simulink library "hvs_framelib_zfCetrax"  (R2016a)
settings: Solver=ode1  StartTime=0.0  StopTime=Inf  FixedStep=0.001  RelTol=1e-3
undefined symbols (not defined in the file): API1_dcac_efficiency, API2_dcac_efficiency, API3_dcac_efficiency, aux_power_flag, aux_power_selector_aux_power_flag, dcdc_effmap, dcdc_effmap_cooltemp_3rdD, dcdc_effmap_cur_2ndD, dcdc_effmap_vlt_1stD, DCL1_dcdc_effmap, DCL1_dcdc_effmap_cooltemp_3rdD, DCL1_dcdc_effmap_cur_2ndD, DCL1_dcdc_effmap_vlt_1stD
libraries: Electrical_to_Mechanical_gen x9, Electrical_converter x6, Electrical_to_Thermal_gen x3, Electrical_charger x3, Powernet x3, Enrg_conv_El_to_Mec_zfCetrax x3, ePTO x3, simulink x3
(part 2 of 2)

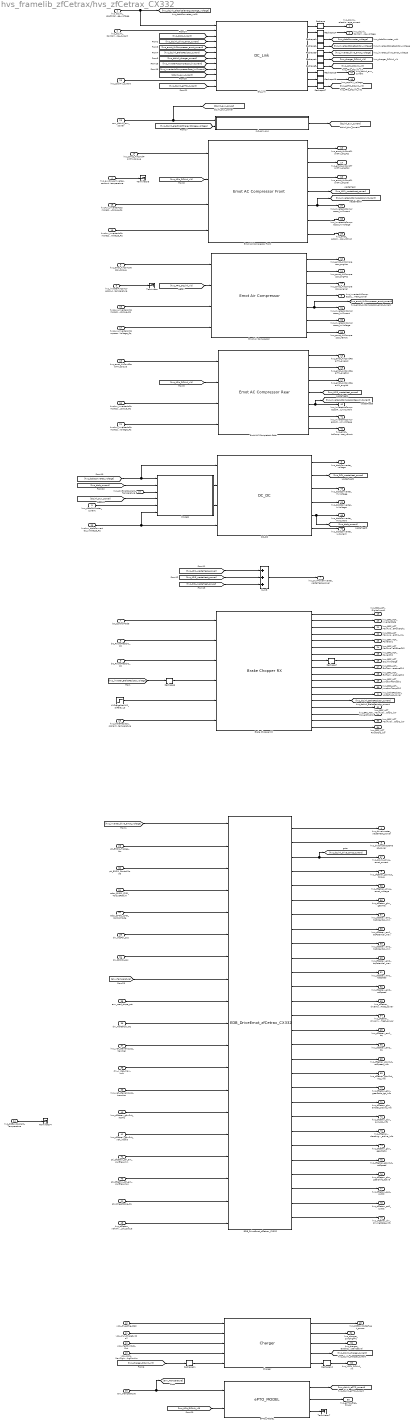
== system hvs_framelib_zfCetrax/hvs_zfCetrax_CX332 ==
  hvs_dcLink_electricalEnergyStorage_voltage : Inport
  hvs_dcLink_ControllableEnergySource_current : Inport  Port=2
  hvs_dcdcConverter_current : Inport  Port=3
  hvs_auxPowerInverter_coolant_temperature : Inport  Port=4
  hvs_inverterAirCompressor_coolant_temperature : Inport  Port=5
  hvs_emot_AirCompressor_torque : Inport  Port=6
  brc_ControlMode : Inport  Port=7
  brc_PowerReqCh1_kW : Inport  Port=8
  brc_PowerReqCh2_kW : Inport  Port=9
  vccu_PlugChrg_Stat : Inport  Port=10
  vccu_Pwr_ChargSysSoll : Inport  Port=11
  vccu_TestPwrSLQ_Out : Inport  Port=12
  vccu_CAN_MaxPlginChrgPwrLim : Inport  Port=13
  hvs_emot_AirCondFrontHV_torque : Inport  Port=14
  hvs_emot_AirCondRearHV_torque : Inport  Port=15
  hvsAux_InverterAirCompressor_torque_Rq : Inport  Port=16
  hvsAux_InverterAirCompressor_Voltage_Rq : Inport  Port=17
  hvsAux_InverterAcCompressorFront_torque_Rq : Inport  Port=18
  hvsAux_InverterAcCompressorFront_Voltage_Rq : Inport  Port=19
  hvsAux_InverterAcCompressorRear_torque_Rq : Inport  Port=20
  hvsAux_InverterAcCompressorRear_Voltage_Rq : Inport  Port=21
  hvsAux_dcdcConverter_LvVoltage_Rq : Inport  Port=22
  env_dcLink_aux_power : Inport  Port=23
  hvs_DCBoxCoolant_Temperature : Inport  Port=24
  hvs_coolHV_current : Inport  Port=25
  env_Temperature : Inport  Port=26
  hvs_drvEmotCoolant_Temperature : Inport  Port=27
  hvs_brakeResistor_coolant_temperature : Inport  Port=28
  pti_EMD1_TrqReq_Nm : Inport  Port=29
  pti_EMD1_ControlMode : Inport  Port=30
  edcu_EMD1_CMD_TorqueRefLim : Inport  Port=31
  edcu_EMD1_CMD_ControlMode : Inport  Port=32
  drv_AccPdl_pos : Inport  Port=33
  drv_BrkPdl_pos : Inport  Port=34
  env_road_slope_pct : Inport  Port=35
  drv_HaltBrkSw_Rq : Inport  Port=36
  hvs_veh_GenericLoss_transVel : Inport  Port=37
  drv_v_des_max_kmh : Inport  Port=38
  hvs_veh_GenericLoss_transAcc : Inport  Port=39
  hvs_zfCetrax_gbxOut_resTrq : Inport  Port=40
  hvs_zfCetrax_gbxOut_veh_inertia : Inport  Port=41
  pti_zfCetrax_ctrl_em_pwrElec_min : Inport  Port=42
  pti_zfCetrax_ctrl_em_pwrElec_max : Inport  Port=43
  pti_WheelBrake_trq : Inport  Port=44
  hvs_zfCetrax_vehWheel_brk_torque : Inport  Port=45
  Brake Chopper RX : Electrical_to_Thermal_gen/Brake Chopper RX
  Charger : Electrical_charger/Charger
  DC_DC : Electrical_converter/DC_DC
  DC_Link : Powernet/DC_Link
  EDB_DriveEmot_zfCetrax_CX332 : Enrg_conv_El_to_Mec_zfCetrax/EDB_DriveEmot_zfCetrax_CX332
  Emot AC Compressor Front : Electrical_to_Mechanical_gen/Emot AC Compressor Front
  Emot AC Compressor Rear : Electrical_to_Mechanical_gen/Emot AC Compressor Rear
  Emot Air Compressor : Electrical_to_Mechanical_gen/Emot Air Compressor
  HVFreigabeHW2_SiRelay_D : Step  Time=5.502  SampleTime=0
  Process : Subsystem
  Reshape{,1..7,11..12,14..17} (14 alike) : Reshape
  Sum8 : Sum  Inputs=+++  SaturateOnIntegerOverflow=on  InputSameDT=on  OutDataTypeStr=Inherit: Same as first input
  Terminator{,4..5,7} (4 alike) : Terminator
  ePTO_MODEL : ePTO/ePTO_MODEL
  sub_env_aux : Subsystem
  hvs_dcLink_electricalEnergyStorage_current : Outport
  hvs_dcLink_ControllableEnergySource_voltage : Outport  Port=2
  hvs_dcdcConverter_voltage : Outport  Port=3
  hvs_driveInverter_wasteHeat_power : Outport  Port=4
  hvs_drvEmotWasteHeat_power : Outport  Port=5
  hvs_brakeResistor_wasteHeat_power : Outport  Port=6
  hvs_auxPowerInverter_wasteHeat_power : Outport  Port=7
  hvs_inverterAirCompressor_wasteHeat_power : Outport  Port=8
  hvs_zfCetrax_gbxOut_torque : Outport  Port=9
  hvs_emot_AirCompressor_angAcc : Outport  Port=10
  hvs_emot_AirCompressor_angPos : Outport  Port=11
  hvs_emot_AirCompressor_angVel : Outport  Port=12
  hvs_emot_AirCondFrontHV_angAcc : Outport  Port=13
  hvs_emot_AirCondFrontHV_angPos : Outport  Port=14
  hvs_emot_AirCondFrontHV_angVel : Outport  Port=15
  hvs_emot_AirCondRearHV_angAcc : Outport  Port=16
  hvs_emot_AirCondRearHV_angVel : Outport  Port=17
  hvs_emot_AirCondRearHV_angPos : Outport  Port=18
  hvs_BRC_ACT_DigitalInput1 : Outport  Port=19
  hvs_BRC_ACT_InverterState : Outport  Port=20
  hvs_BRC_ACT_MaxAvailablePowerCh1 : Outport  Port=21
  hvs_BRC_ACT_MaxAvailablePowerCh1_VAL : Outport  Port=22
  hvs_BRC_ACT_PowerCh1 : Outport  Port=23
  hvs_BRC_ACT_MaxAvailablePowerCh2 : Outport  Port=24
  hvs_BRC_ACT_PowerCh2 : Outport  Port=25
  hvs_BRC_ACT_DcLinkVoltage : Outport  Port=26
  hvs_BRC_ACT_ExtTemperatureCh1 : Outport  Port=27
  hvs_BRC_ACT_ExtTemperatureCh2 : Outport  Port=28
  hvs_BRC_ACT_JunctionTempCh1 : Outport  Port=29
  hvs_BRC_ACT_JunctionTempCh2 : Outport  Port=30
  hvs_charger_pwrChrgPhy : Outport  Port=31
  hvs_charger_ExtChrgr_Isolation_ResistanceCval : Outport  Port=32
  hvs_VCCU_DCLink_vlt : Outport  Port=33
  hvs_InverterAirCompressor_hvCurrent : Outport  Port=34
  hvs_InverterAirCompressor_hvVoltage : Outport  Port=35
  hvs_emot_AirCompressor_nEmot : Outport  Port=36
  hvs_InverterAcCompressor_hvCurrent : Outport  Port=37
  hvs_InverterAcCompressor_hvVoltage : Outport  Port=38
  hvs_emot_AcCompressor_nEmot : Outport  Port=39
  hvs_InverterAcCompressorRear_hvCurrent : Outport  Port=40
  hvs_InverterAcCompressorRear_hvVoltage : Outport  Port=41
  hvs_emot_AcCompressorRear_nEmot : Outport  Port=42
  hvs_dcdcConverter_HvVoltage : Outport  Port=43
  hvs_dcdcConverter_LvVoltage : Outport  Port=44
  hvs_dcdcConverter_HvCurrent : Outport  Port=45
  hvs_dcdcConverter_LvCurrent : Outport  Port=46
  hvs_dcLink_aux_current : Outport  Port=47
  hvs_DCBoxWasteHeat_power : Outport  Port=48
  hvs_coolHV_voltage : Outport  Port=49
  hvs_ePTO_Elec_Power : Outport  Port=50
  hvs_BRC_ACT_MaxAvailablePowerCh1_kW : Outport  Port=51
  hvs_BRC_ACT_PowerCh1_kW : Outport  Port=52
  hvs_BRC_ACT_MaxAvailablePowerCh2_kW : Outport  Port=53
  hvs_BRC_ACT_PowerCh2_kW : Outport  Port=54
  hvs_zfCetrax_drive_emot_voltage : Outport  Port=55
  hvs_zfCetrax_gbx_gearAct : Outport  Port=56
  hvs_zfCetrax_em1_trqPotential_min : Outport  Port=57
  hvs_zfCetrax_em1_trqPotential_max : Outport  Port=58
  hvs_zfCetrax_em2_trqPotential_min : Outport  Port=59
  hvs_zfCetrax_em2_trqPotential_max : Outport  Port=60
  hvs_zfCetrax_em1_rotSpeed : Outport  Port=61
  hvs_zfCetrax_em2_rotSpeed : Outport  Port=62
  hvs_zfCetrax_drvEmotWasteHeat_power : Outport  Port=63
  hvs_zfCetrax_driveInverterWasteHeat_power : Outport  Port=64
  hvs_zfCetrax_em1_trq : Outport  Port=65
  hvs_zfCetrax_em2_trq : Outport  Port=66
  hvs_dcLink_drive_emot_current : Outport  Port=67
  hvs_zfCetrax_gbxOut_rotSpeed_info : Outport  Port=68
  hvs_zfCetrax_gbxOut_Acc_info : Outport  Port=69
  hvs_zfCetrax_gbx_gearRatio_tgt_info : Outport  Port=70
  hvs_zfCetrax_gbx_emDec_active_info : Outport  Port=71
  hvs_zfCetrax_gbx_pwrLoss_info : Outport  Port=72
  hvs_zfCetrax_derating_active_info : Outport  Port=73
  hvs_zfCetrax_gbx_gearRatio : Outport  Port=74
  hvs_zfCetrax_gbxOut_rotSpeed : Outport  Port=75
  hvs_zfCetrax_gbx_gearShift_active : Outport  Port=76
  hvs_zfCetrax_pe1_curDC : Outport  Port=77
  hvs_zfCetrax_pe2_curDC : Outport  Port=78
  hvs_zfCetrax_drv_drivingState_info : Outport  Port=79
  wires:
  EDB_DriveEmot_zfCetrax_CX332/28 -> hvs_zfCetrax_drv_drivingState_info/1
  Process/2(hvs_dcdcConv_current1) -> DC_DC/3
  Process/1(dcdc_conv_eff) -> DC_DC/2
  hvs_dcdcConverter_current/1 -> Process/5(hvs_dcdcConv_current)
  [dcLink_aux_power] -> Process/4(dcLink_aux_power)  "dcLink_aux_power"
  hvs_drvEmotCoolant_Temperature/1 -> Process/3(hvs_drvEmotCoolant_Temperature)
  [hvs_dcdc_current] -> Process/2(hvs_dcdc_HvCurrent)  "hvs_dcdc_HvCurrent"
  [hvs_dcLink_ePTO_current] -> DC_Link/12
  [hvs_APIs_DCLink_vlt] -> ePTO_MODEL/2
  ePTO_MODEL/3 -> Terminator7/1
  ePTO_MODEL/2 -> hvs_ePTO_Elec_Power/1
  ePTO_MODEL/1 -> [hvs_dcLink_ePTO_current]
  DC_Link/10 -> Reshape17/1
  Reshape17/1 -> [hvs_ePTO_DCLink_vlt]
  env_Temperature/1 -> [env_Temperature], ePTO_MODEL/1
  hvs_DCBoxCoolant_Temperature/1 -> Terminator4/1
  Charger/1 -> hvs_DCBoxWasteHeat_power/1  "hvs_DCBoxWasteHeat_power"
  hvsAux_dcdcConverter_LvVoltage_Rq/1 -> DC_DC/4, Process/6(hvsAux_dcdcConv_LvVoltage_Rq)  "hvsAux_dcdcConverter_LvVoltage_Rq"
  DC_Link/8 -> Reshape15/1
  [hvs_dcLink_electricalEnergyStorage_voltage] -> sub_env_aux/2(Nebenagg_voltage)
  sub_env_aux/1(dcLink_aux_current) -> [dcLink_aux_current]
  env_dcLink_aux_power/1 -> sub_env_aux/1(env_dcLink_aux_power), [dcLink_aux_power]
  [dcLink_aux_current] -> DC_Link/10
  Reshape12/1 -> hvs_VCCU_DCLink_vlt/1
  Reshape11/1 -> Charger/5
  Reshape7/1 -> hvs_BRC_ACT_DcLinkVoltage/1
  Reshape6/1 -> Brake Chopper RX/4
  Reshape5/1 -> [hvs_APIs_DCLink_vlt]
  Reshape4/1 -> [hvs_charger_DCLink_vlt]
  Reshape3/1 -> [hvs_inverter_drive_emot_voltage]
  Reshape2/1 -> [hvs_inverter_BrakeResistor_voltage]
  Reshape1/1 -> [hvs_dcdcConverter_voltage]
  Reshape/1 -> hvs_dcLink_electricalEnergyStorage_current/1
  [hvs_dcdc_current] -> DC_Link/3
  [hvs_DCL_wasteHeat_power] -> Sum8/3
  [hvs_API3_wasteHeat_power] -> Sum8/2
  [hvs_API1_wasteHeat_power] -> Sum8/1
  Sum8/1 -> hvs_auxPowerInverter_wasteHeat_power/1
  DC_DC/6 -> hvs_dcdcConverter_LvCurrent/1
  DC_DC/5 -> hvs_dcdcConverter_HvCurrent/1, [hvs_dcdc_current]
  DC_DC/4 -> hvs_dcdcConverter_LvVoltage/1
  DC_DC/3 -> hvs_dcdcConverter_HvVoltage/1
  DC_Link/3 -> Reshape1/1
  DC_DC/1 -> hvs_dcdcConverter_voltage/1
  DC_DC/2 -> [hvs_DCL_wasteHeat_power]
  [hvs_dcdcConverter_voltage] -> Process/1(hvs_dcdcConverter_voltage), DC_DC/1  "hvs_dcdcConverter_voltage"
  Emot AC Compressor Rear/4 -> [hvs_API3_wasteHeat_power]
  Emot AC Compressor Rear/5 -> hvs_InverterAcCompressorRear_hvCurrent/1, [hvs_InverterAcCompressorRear_hvCurrent]
  Emot AC Compressor Rear/6 -> hvs_InverterAcCompressorRear_hvVoltage/1
  Emot AC Compressor Rear/7 -> hvs_emot_AcCompressorRear_nEmot/1
  Emot AC Compressor Rear/2 -> hvs_emot_AirCondRearHV_angPos/1
  Emot AC Compressor Rear/3 -> hvs_emot_AirCondRearHV_angVel/1
  Emot AC Compressor Rear/1 -> hvs_emot_AirCondRearHV_angAcc/1
  hvsAux_InverterAcCompressorRear_Voltage_Rq/1 -> Emot AC Compressor Rear/4
  hvsAux_InverterAcCompressorRear_torque_Rq/1 -> Emot AC Compressor Rear/3
  [hvs_APIs_DCLink_vlt] -> Emot AC Compressor Rear/2
  hvs_emot_AirCondRearHV_torque/1 -> Emot AC Compressor Rear/1
  Emot AC Compressor Front/4 -> [hvs_API1_wasteHeat_power]
  Emot AC Compressor Front/6 -> hvs_InverterAcCompressor_hvVoltage/1
  Emot AC Compressor Front/7 -> hvs_emot_AcCompressor_nEmot/1
  Emot AC Compressor Front/3 -> hvs_emot_AirCondFrontHV_angVel/1
  Emot AC Compressor Front/2 -> hvs_emot_AirCondFrontHV_angPos/1
  Emot AC Compressor Front/1 -> hvs_emot_AirCondFrontHV_angAcc/1
  hvsAux_InverterAcCompressorFront_Voltage_Rq/1 -> Emot AC Compressor Front/4
  hvsAux_InverterAcCompressorFront_torque_Rq/1 -> Emot AC Compressor Front/3
  hvs_emot_AirCondFrontHV_torque/1 -> Emot AC Compressor Front/1
  [hvs_APIs_DCLink_vlt] -> Emot AC Compressor Front/2
  hvs_auxPowerInverter_coolant_temperature/1 -> Terminator5/1
  hvs_inverterAirCompressor_coolant_temperature/1 -> Terminator/1
  hvsAux_InverterAirCompressor_Voltage_Rq/1 -> Emot Air Compressor/4
  hvsAux_InverterAirCompressor_torque_Rq/1 -> Emot Air Compressor/3
  [hvs_APIs_DCLink_vlt] -> Emot Air Compressor/2
  DC_Link/7 -> Reshape5/1
  Emot Air Compressor/6 -> hvs_InverterAirCompressor_hvVoltage/1
  Emot Air Compressor/7 -> hvs_emot_AirCompressor_nEmot/1
  Emot Air Compressor/5 -> [hvs_emot_AirCompressor_emot_current], hvs_InverterAirCompressor_hvCurrent/1
  Emot Air Compressor/4 -> hvs_inverterAirCompressor_wasteHeat_power/1
  Emot Air Compressor/3 -> hvs_emot_AirCompressor_angVel/1
  Emot Air Compressor/2 -> hvs_emot_AirCompressor_angPos/1
  Emot Air Compressor/1 -> hvs_emot_AirCompressor_angAcc/1
  hvs_emot_AirCompressor_torque/1 -> Emot Air Compressor/1
  DC_Link/1 -> Reshape/1
  DC_Link/2 -> Reshape14/1
  hvs_dcLink_electricalEnergyStorage_voltage/1 -> [hvs_dcLink_electricalEnergyStorage_voltage], DC_Link/1
  hvs_dcLink_ControllableEnergySource_current/1 -> DC_Link/2
  DC_Link/4 -> Reshape2/1
  Brake Chopper RX/1 -> hvs_BRC_ACT_DigitalInput1/1
  Brake Chopper RX/2 -> hvs_BRC_ACT_InverterState/1
  Brake Chopper RX/3 -> hvs_BRC_ACT_MaxAvailablePowerCh1/1
  Brake Chopper RX/4 -> hvs_BRC_ACT_MaxAvailablePowerCh1_VAL/1
  Brake Chopper RX/5 -> hvs_BRC_ACT_PowerCh1/1
  Brake Chopper RX/6 -> hvs_BRC_ACT_MaxAvailablePowerCh2/1
  Brake Chopper RX/7 -> hvs_BRC_ACT_PowerCh2/1
  Brake Chopper RX/8 -> Reshape7/1
  Brake Chopper RX/9 -> hvs_BRC_ACT_ExtTemperatureCh1/1
  Brake Chopper RX/10 -> hvs_BRC_ACT_ExtTemperatureCh2/1
  Brake Chopper RX/11 -> hvs_BRC_ACT_JunctionTempCh1/1
  Brake Chopper RX/12 -> hvs_BRC_ACT_JunctionTempCh2/1
  [hvs_inverter_BrakeResistor_voltage] -> Reshape6/1
  DC_Link/5 -> Reshape3/1
  [hvs_dcLink_drive_emot_current] -> DC_Link/4
  [hvs_emot_AirCompressor_emot_current] -> DC_Link/5
  Brake Chopper RX/13 -> hvs_brakeResistor_wasteHeat_power/1
  Brake Chopper RX/14 -> [hvs_dcLink_BrakeResistor_current]
  [hvs_dcLink_BrakeResistor_current] -> DC_Link/6
  vccu_CAN_MaxPlginChrgPwrLim/1 -> Charger/4
  [hvs_charger_DCLink_vlt] -> Reshape11/1
  vccu_TestPwrSLQ_Out/1 -> Charger/3
  vccu_Pwr_ChargSysSoll/1 -> Charger/2
  vccu_PlugChrg_Stat/1 -> Charger/1
  Charger/2 -> hvs_charger_pwrChrgPhy/1
  Charger/3 -> hvs_charger_ExtChrgr_Isolation_ResistanceCval/1
  Charger/4 -> [hvs_dcLink_charger_current]
  [hvs_dcLink_charger_current] -> DC_Link/7
  DC_Link/6 -> Reshape4/1
  Charger/5 -> Reshape12/1
  Emot AC Compressor Front/5 -> [hvs_InverterAcCompressor_hvCurrent], hvs_InverterAcCompressor_hvCurrent/1
  [hvs_InverterAcCompressor_hvCurrent] -> DC_Link/8
  [hvs_InverterAcCompressorRear_hvCurrent] -> DC_Link/9
  Reshape14/1 -> hvs_dcLink_ControllableEnergySource_voltage/1
  Reshape15/1 -> hvs_dcLink_aux_current/1
  DC_Link/9 -> Reshape16/1
  Reshape16/1 -> hvs_coolHV_voltage/1
  hvs_coolHV_current/1 -> DC_Link/11
  HVFreigabeHW2_SiRelay_D/1 -> Brake Chopper RX/5
  brc_ControlMode/1 -> Brake Chopper RX/1
  brc_PowerReqCh1_kW/1 -> Brake Chopper RX/2
  brc_PowerReqCh2_kW/1 -> Brake Chopper RX/3
  hvs_brakeResistor_coolant_temperature/1 -> Brake Chopper RX/6
  Brake Chopper RX/15 -> hvs_BRC_ACT_MaxAvailablePowerCh1_kW/1
  Brake Chopper RX/16 -> hvs_BRC_ACT_PowerCh1_kW/1
  Brake Chopper RX/17 -> hvs_BRC_ACT_MaxAvailablePowerCh2_kW/1
  Brake Chopper RX/18 -> hvs_BRC_ACT_PowerCh2_kW/1
  [hvs_inverter_drive_emot_voltage] -> EDB_DriveEmot_zfCetrax_CX332/1
  pti_EMD1_TrqReq_Nm/1 -> EDB_DriveEmot_zfCetrax_CX332/2
  pti_EMD1_ControlMode/1 -> EDB_DriveEmot_zfCetrax_CX332/3
  edcu_EMD1_CMD_TorqueRefLim/1 -> EDB_DriveEmot_zfCetrax_CX332/4
  edcu_EMD1_CMD_ControlMode/1 -> EDB_DriveEmot_zfCetrax_CX332/5
  drv_AccPdl_pos/1 -> EDB_DriveEmot_zfCetrax_CX332/6
  drv_BrkPdl_pos/1 -> EDB_DriveEmot_zfCetrax_CX332/7
  [env_Temperature] -> EDB_DriveEmot_zfCetrax_CX332/8
  env_road_slope_pct/1 -> EDB_DriveEmot_zfCetrax_CX332/9
  drv_HaltBrkSw_Rq/1 -> EDB_DriveEmot_zfCetrax_CX332/10
  hvs_veh_GenericLoss_transVel/1 -> EDB_DriveEmot_zfCetrax_CX332/11
  drv_v_des_max_kmh/1 -> EDB_DriveEmot_zfCetrax_CX332/12
  hvs_veh_GenericLoss_transAcc/1 -> EDB_DriveEmot_zfCetrax_CX332/13
  hvs_zfCetrax_gbxOut_resTrq/1 -> EDB_DriveEmot_zfCetrax_CX332/14
  hvs_zfCetrax_gbxOut_veh_inertia/1 -> EDB_DriveEmot_zfCetrax_CX332/15
  pti_zfCetrax_ctrl_em_pwrElec_min/1 -> EDB_DriveEmot_zfCetrax_CX332/16
  pti_zfCetrax_ctrl_em_pwrElec_max/1 -> EDB_DriveEmot_zfCetrax_CX332/17
  EDB_DriveEmot_zfCetrax_CX332/3 -> hvs_dcLink_drive_emot_current/1, [hvs_dcLink_drive_emot_current]
  EDB_DriveEmot_zfCetrax_CX332/1 -> hvs_driveInverter_wasteHeat_power/1
  EDB_DriveEmot_zfCetrax_CX332/2 -> hvs_drvEmotWasteHeat_power/1
  EDB_DriveEmot_zfCetrax_CX332/4 -> hvs_zfCetrax_gbxOut_torque/1
  EDB_DriveEmot_zfCetrax_CX332/5 -> hvs_zfCetrax_drive_emot_voltage/1
  EDB_DriveEmot_zfCetrax_CX332/6 -> hvs_zfCetrax_gbx_gearAct/1
  EDB_DriveEmot_zfCetrax_CX332/7 -> hvs_zfCetrax_em1_trqPotential_min/1
  EDB_DriveEmot_zfCetrax_CX332/8 -> hvs_zfCetrax_em1_trqPotential_max/1
  EDB_DriveEmot_zfCetrax_CX332/9 -> hvs_zfCetrax_em2_trqPotential_min/1
  EDB_DriveEmot_zfCetrax_CX332/10 -> hvs_zfCetrax_em2_trqPotential_max/1
  EDB_DriveEmot_zfCetrax_CX332/11 -> hvs_zfCetrax_em1_rotSpeed/1
  EDB_DriveEmot_zfCetrax_CX332/12 -> hvs_zfCetrax_em2_rotSpeed/1
  EDB_DriveEmot_zfCetrax_CX332/13 -> hvs_zfCetrax_drvEmotWasteHeat_power/1
  EDB_DriveEmot_zfCetrax_CX332/14 -> hvs_zfCetrax_driveInverterWasteHeat_power/1
  EDB_DriveEmot_zfCetrax_CX332/15 -> hvs_zfCetrax_em1_trq/1
  EDB_DriveEmot_zfCetrax_CX332/16 -> hvs_zfCetrax_em2_trq/1
  pti_WheelBrake_trq/1 -> EDB_DriveEmot_zfCetrax_CX332/18
  EDB_DriveEmot_zfCetrax_CX332/17 -> hvs_zfCetrax_gbxOut_rotSpeed_info/1
  EDB_DriveEmot_zfCetrax_CX332/18 -> hvs_zfCetrax_gbxOut_Acc_info/1
  EDB_DriveEmot_zfCetrax_CX332/19 -> hvs_zfCetrax_gbx_gearRatio_tgt_info/1
  EDB_DriveEmot_zfCetrax_CX332/20 -> hvs_zfCetrax_gbx_emDec_active_info/1
  EDB_DriveEmot_zfCetrax_CX332/21 -> hvs_zfCetrax_gbx_pwrLoss_info/1
  EDB_DriveEmot_zfCetrax_CX332/22 -> hvs_zfCetrax_derating_active_info/1
  EDB_DriveEmot_zfCetrax_CX332/23 -> hvs_zfCetrax_gbx_gearRatio/1
  hvs_zfCetrax_vehWheel_brk_torque/1 -> EDB_DriveEmot_zfCetrax_CX332/19
  EDB_DriveEmot_zfCetrax_CX332/24 -> hvs_zfCetrax_gbxOut_rotSpeed/1
  EDB_DriveEmot_zfCetrax_CX332/25 -> hvs_zfCetrax_gbx_gearShift_active/1
  EDB_DriveEmot_zfCetrax_CX332/26 -> hvs_zfCetrax_pe1_curDC/1
  EDB_DriveEmot_zfCetrax_CX332/27 -> hvs_zfCetrax_pe2_curDC/1

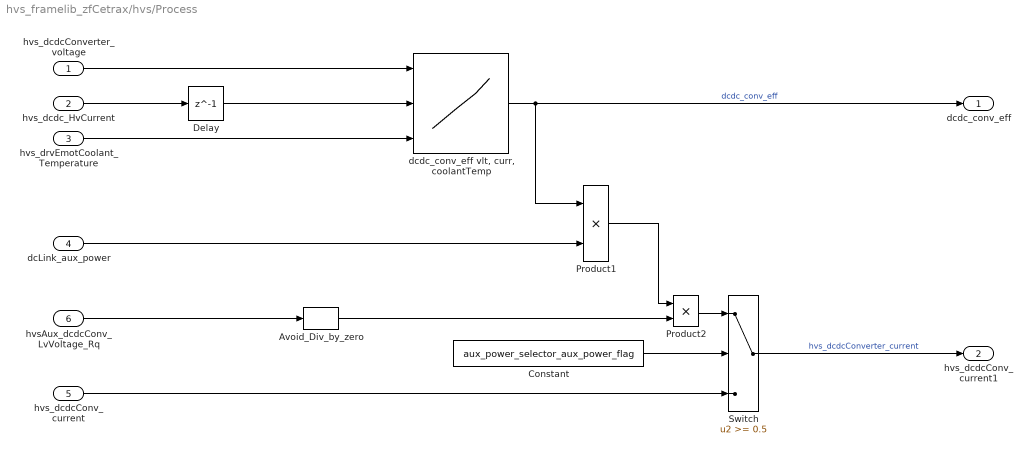
== system hvs_framelib_zfCetrax/hvs/Process ==
  hvs_dcdcConverter_voltage : Inport
  hvs_dcdc_HvCurrent : Inport  Port=2
  hvs_drvEmotCoolant_Temperature : Inport  Port=3
  dcLink_aux_power : Inport  Port=4
  hvs_dcdcConv_current : Inport  Port=5
  hvsAux_dcdcConv_LvVoltage_Rq : Inport  Port=6
  Avoid_Div_by_zero : Electrical_converter/DC_DC/Avoid_Div_by_zero
  Constant : Constant  Value=aux_power_selector_aux_power_flag
  Delay : Delay  DelayLength=1  InitialCondition=0
  Product1 : Product  Inputs=**  RndMeth=Zero
  Product2 : Product  Inputs=**  RndMeth=Zero
  Switch : Switch  Threshold=0.5
  "dcdc_conv_eff vlt, curr, coolantTemp" : Lookup_n-D  NumberOfTableDimensions=3  BreakpointsForDimension1=DCL1_dcdc_effmap_vlt_1stD  BreakpointsForDimension2=DCL1_dcdc_effmap_cur_2ndD  BreakpointsForDimension3=DCL1_dcdc_effmap_cooltemp_3rdD  Table=DCL1_dcdc_effmap  ExtrapMethod=Clip  RndMeth=Simplest  InputSameDT=on
  dcdc_conv_eff : Outport
  hvs_dcdcConv_current1 : Outport  Port=2
  wires:
  Delay/1 -> "dcdc_conv_eff vlt, curr, coolantTemp"/2
  hvs_dcdc_HvCurrent/1 -> Delay/1
  "dcdc_conv_eff vlt, curr, coolantTemp"/1 -> dcdc_conv_eff/1, Product1/1  "dcdc_conv_eff"
  Product2/1 -> Switch/1
  Product1/1 -> Product2/1
  hvs_dcdcConv_current/1 -> Switch/3
  Switch/1 -> hvs_dcdcConv_current1/1  "hvs_dcdcConverter_current"
  dcLink_aux_power/1 -> Product1/2
  Avoid_Div_by_zero/1 -> Product2/2
  Constant/1 -> Switch/2
  hvsAux_dcdcConv_LvVoltage_Rq/1 -> Avoid_Div_by_zero/1
  hvs_dcdcConverter_voltage/1 -> "dcdc_conv_eff vlt, curr, coolantTemp"/1
  hvs_drvEmotCoolant_Temperature/1 -> "dcdc_conv_eff vlt, curr, coolantTemp"/3

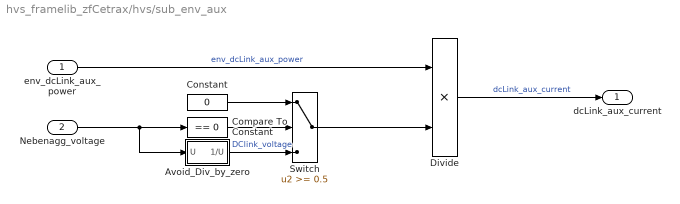
== system hvs_framelib_zfCetrax/hvs/sub_env_aux ==
  env_dcLink_aux_power : Inport
  Nebenagg_voltage : Inport  Port=2
  Avoid_Div_by_zero : Subsystem
  Compare To Constant : simulink/Logic and Bit Operations/Compare To Constant  relop===  const=0  OutDataTypeStr=boolean
  Constant : Constant  Value=0
  Divide : Product
  Switch : Switch  Threshold=0.5
  dcLink_aux_current : Outport
  wires:
  Divide/1 -> dcLink_aux_current/1  "dcLink_aux_current"
  Nebenagg_voltage/1 -> Avoid_Div_by_zero/1(U), Compare To Constant/1
  Avoid_Div_by_zero/1(1/U) -> Switch/3  "DClink_voltage"
  env_dcLink_aux_power/1 -> Divide/1  "env_dcLink_aux_power"
  Compare To Constant/1 -> Switch/2
  Constant/1 -> Switch/1
  Switch/1 -> Divide/2

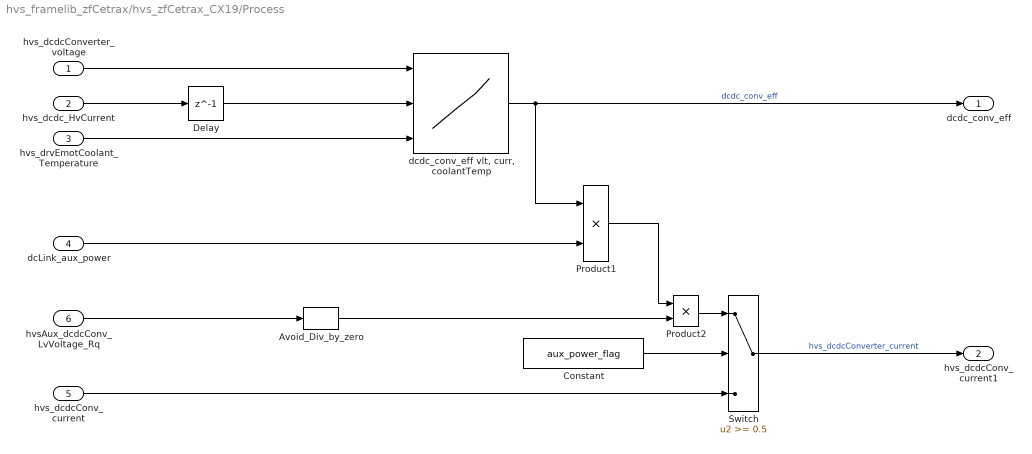
== system hvs_framelib_zfCetrax/hvs_zfCetrax_CX19/Process ==
  hvs_dcdcConverter_voltage : Inport
  hvs_dcdc_HvCurrent : Inport  Port=2
  hvs_drvEmotCoolant_Temperature : Inport  Port=3
  dcLink_aux_power : Inport  Port=4
  hvs_dcdcConv_current : Inport  Port=5
  hvsAux_dcdcConv_LvVoltage_Rq : Inport  Port=6
  Avoid_Div_by_zero : Electrical_converter/DC_DC/Avoid_Div_by_zero
  Constant : Constant  Value=aux_power_flag
  Delay : Delay  DelayLength=1  InitialCondition=0
  Product1 : Product  Inputs=**  RndMeth=Zero
  Product2 : Product  Inputs=**  RndMeth=Zero
  Switch : Switch  Threshold=0.5
  "dcdc_conv_eff vlt, curr, coolantTemp" : Lookup_n-D  NumberOfTableDimensions=3  BreakpointsForDimension1=dcdc_effmap_vlt_1stD  BreakpointsForDimension2=dcdc_effmap_cur_2ndD  BreakpointsForDimension3=dcdc_effmap_cooltemp_3rdD  Table=dcdc_effmap  ExtrapMethod=Clip  RndMeth=Simplest  InputSameDT=on
  dcdc_conv_eff : Outport
  hvs_dcdcConv_current1 : Outport  Port=2
  wires:
  hvs_drvEmotCoolant_Temperature/1 -> "dcdc_conv_eff vlt, curr, coolantTemp"/3
  hvs_dcdcConverter_voltage/1 -> "dcdc_conv_eff vlt, curr, coolantTemp"/1
  hvsAux_dcdcConv_LvVoltage_Rq/1 -> Avoid_Div_by_zero/1
  Constant/1 -> Switch/2
  Avoid_Div_by_zero/1 -> Product2/2
  dcLink_aux_power/1 -> Product1/2
  Switch/1 -> hvs_dcdcConv_current1/1  "hvs_dcdcConverter_current"
  hvs_dcdcConv_current/1 -> Switch/3
  Product1/1 -> Product2/1
  Product2/1 -> Switch/1
  "dcdc_conv_eff vlt, curr, coolantTemp"/1 -> Product1/1, dcdc_conv_eff/1  "dcdc_conv_eff"
  hvs_dcdc_HvCurrent/1 -> Delay/1
  Delay/1 -> "dcdc_conv_eff vlt, curr, coolantTemp"/2

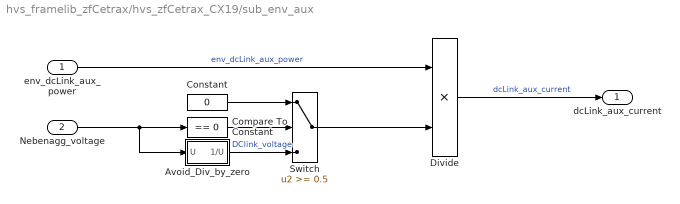
== system hvs_framelib_zfCetrax/hvs_zfCetrax_CX19/sub_env_aux ==
  env_dcLink_aux_power : Inport
  Nebenagg_voltage : Inport  Port=2
  Avoid_Div_by_zero : Subsystem
  Compare To Constant : simulink/Logic and Bit Operations/Compare To Constant  relop===  const=0  OutDataTypeStr=boolean
  Constant : Constant  Value=0
  Divide : Product
  Switch : Switch  Threshold=0.5
  dcLink_aux_current : Outport
  wires:
  Switch/1 -> Divide/2
  Constant/1 -> Switch/1
  Compare To Constant/1 -> Switch/2
  env_dcLink_aux_power/1 -> Divide/1  "env_dcLink_aux_power"
  Avoid_Div_by_zero/1(1/U) -> Switch/3  "DClink_voltage"
  Nebenagg_voltage/1 -> Compare To Constant/1, Avoid_Div_by_zero/1(U)
  Divide/1 -> dcLink_aux_current/1  "dcLink_aux_current"

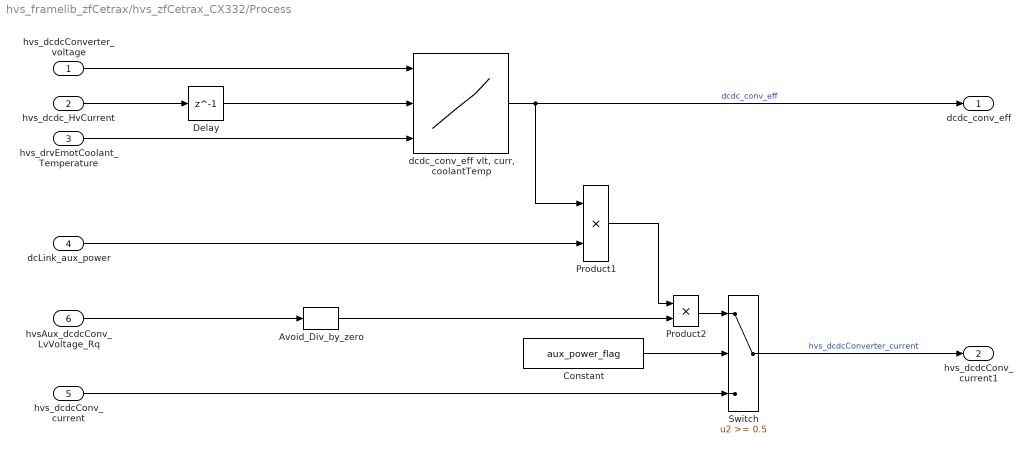
== system hvs_framelib_zfCetrax/hvs_zfCetrax_CX332/Process ==
  hvs_dcdcConverter_voltage : Inport
  hvs_dcdc_HvCurrent : Inport  Port=2
  hvs_drvEmotCoolant_Temperature : Inport  Port=3
  dcLink_aux_power : Inport  Port=4
  hvs_dcdcConv_current : Inport  Port=5
  hvsAux_dcdcConv_LvVoltage_Rq : Inport  Port=6
  Avoid_Div_by_zero : Electrical_converter/DC_DC/Avoid_Div_by_zero
  Constant : Constant  Value=aux_power_flag
  Delay : Delay  DelayLength=1  InitialCondition=0
  Product1 : Product  Inputs=**  RndMeth=Zero
  Product2 : Product  Inputs=**  RndMeth=Zero
  Switch : Switch  Threshold=0.5
  "dcdc_conv_eff vlt, curr, coolantTemp" : Lookup_n-D  NumberOfTableDimensions=3  BreakpointsForDimension1=dcdc_effmap_vlt_1stD  BreakpointsForDimension2=dcdc_effmap_cur_2ndD  BreakpointsForDimension3=dcdc_effmap_cooltemp_3rdD  Table=dcdc_effmap  ExtrapMethod=Clip  RndMeth=Simplest  InputSameDT=on
  dcdc_conv_eff : Outport
  hvs_dcdcConv_current1 : Outport  Port=2
  wires:
  Delay/1 -> "dcdc_conv_eff vlt, curr, coolantTemp"/2
  hvs_dcdc_HvCurrent/1 -> Delay/1
  "dcdc_conv_eff vlt, curr, coolantTemp"/1 -> dcdc_conv_eff/1, Product1/1  "dcdc_conv_eff"
  Product2/1 -> Switch/1
  Product1/1 -> Product2/1
  hvs_dcdcConv_current/1 -> Switch/3
  Switch/1 -> hvs_dcdcConv_current1/1  "hvs_dcdcConverter_current"
  dcLink_aux_power/1 -> Product1/2
  Avoid_Div_by_zero/1 -> Product2/2
  Constant/1 -> Switch/2
  hvsAux_dcdcConv_LvVoltage_Rq/1 -> Avoid_Div_by_zero/1
  hvs_dcdcConverter_voltage/1 -> "dcdc_conv_eff vlt, curr, coolantTemp"/1
  hvs_drvEmotCoolant_Temperature/1 -> "dcdc_conv_eff vlt, curr, coolantTemp"/3

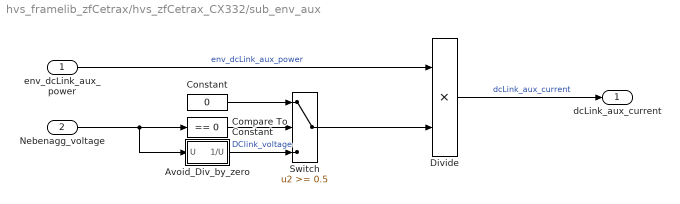
== system hvs_framelib_zfCetrax/hvs_zfCetrax_CX332/sub_env_aux ==
  env_dcLink_aux_power : Inport
  Nebenagg_voltage : Inport  Port=2
  Avoid_Div_by_zero : Subsystem
  Compare To Constant : simulink/Logic and Bit Operations/Compare To Constant  relop===  const=0  OutDataTypeStr=boolean
  Constant : Constant  Value=0
  Divide : Product
  Switch : Switch  Threshold=0.5
  dcLink_aux_current : Outport
  wires:
  Divide/1 -> dcLink_aux_current/1  "dcLink_aux_current"
  Nebenagg_voltage/1 -> Avoid_Div_by_zero/1(U), Compare To Constant/1
  Avoid_Div_by_zero/1(1/U) -> Switch/3  "DClink_voltage"
  env_dcLink_aux_power/1 -> Divide/1  "env_dcLink_aux_power"
  Compare To Constant/1 -> Switch/2
  Constant/1 -> Switch/1
  Switch/1 -> Divide/2

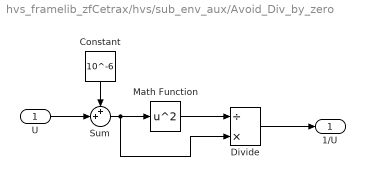
== system hvs_framelib_zfCetrax/hvs/sub_env_aux/Avoid_Div_by_zero ==
  U : Inport
  Constant : Constant  Value=10^-6
  Divide : Product  Inputs=/*
  Math Function : Math  Operator=square  SaturateOnIntegerOverflow=on
  Sum : Sum  Inputs=++|
  1/U : Outport
  wires:
  U/1 -> Sum/2
  Constant/1 -> Sum/1
  Sum/1 -> Math Function/1, Divide/2
  Math Function/1 -> Divide/1
  Divide/1 -> 1/U/1

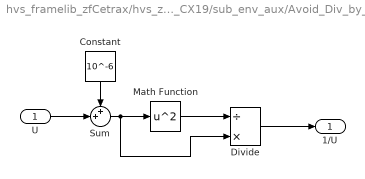
== system hvs_framelib_zfCetrax/hvs_zfCetrax_CX19/sub_env_aux/Avoid_Div_by_zero ==
  U : Inport
  Constant : Constant  Value=10^-6
  Divide : Product  Inputs=/*
  Math Function : Math  Operator=square  SaturateOnIntegerOverflow=on
  Sum : Sum  Inputs=++|
  1/U : Outport
  wires:
  Divide/1 -> 1/U/1
  Math Function/1 -> Divide/1
  Sum/1 -> Divide/2, Math Function/1
  Constant/1 -> Sum/1
  U/1 -> Sum/2

== system hvs_framelib_zfCetrax/hvs_zfCetrax_CX332/sub_env_aux/Avoid_Div_by_zero ==
  U : Inport
  Constant : Constant  Value=10^-6
  Divide : Product  Inputs=/*
  Math Function : Math  Operator=square  SaturateOnIntegerOverflow=on
  Sum : Sum  Inputs=++|
  1/U : Outport
  wires:
  U/1 -> Sum/2
  Constant/1 -> Sum/1
  Sum/1 -> Math Function/1, Divide/2
  Math Function/1 -> Divide/1
  Divide/1 -> 1/U/1
